simulink model "VehicleBackKin"  (R2024b)
settings: Solver=FixedStepAuto  StartTime=0.0  StopTime=inf  FixedStep=VehicleEnv.Ts  RelTol=1e-3
values from neighbouring files (symbols this model uses):
  em = ElectricMotor    [VehicleBackKinEnv.m]
  ess = VehicleEnv.ess    [VehicleBackKinEnv.m]
  fd = FinalDrive    [VehicleBackKinEnv.m]
  gb = Gearbox    [VehicleBackKinEnv.m]
  ice = Engine    [VehicleBackKinEnv.m]
  reward = VehicleEnv.reward    [VehicleBackKinEnv.m]
  selector_in = zeros(size(obs_info.Name))    [VehicleBackKinEnv.m]
  veh = Vehicle    [VehicleBackKinEnv.m]
  VehicleEnv = evalin("base","VehicleEnv")    [VehicleBackKinEnv.m]
  wh = Wheels    [VehicleBackKinEnv.m]
undefined symbols (not defined in the file or in its folder): agentSampleTime, cycle_insimulink, cycleTime, transfer_fun_coeff
libraries: simulink x3, rllib x1, autolibsharedcoreengin x1
(part 1 of 4)
settings Model: PauseTimes=144  Creator=d043083  LastModifiedBy=d043083
settings SolverCC: ZeroCrossAlgorithm=Adaptive
settings DebuggingCC: IgnoredZcDiagnostic=none
settings RTWCC: GPUComputeCapability=3.5

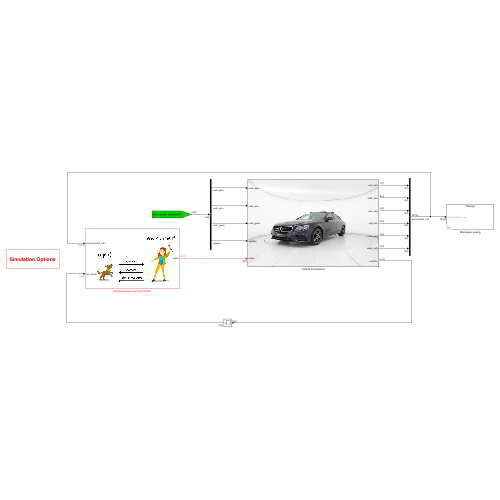
[thumbnail: Simulink's stored preview of the top-level diagram]
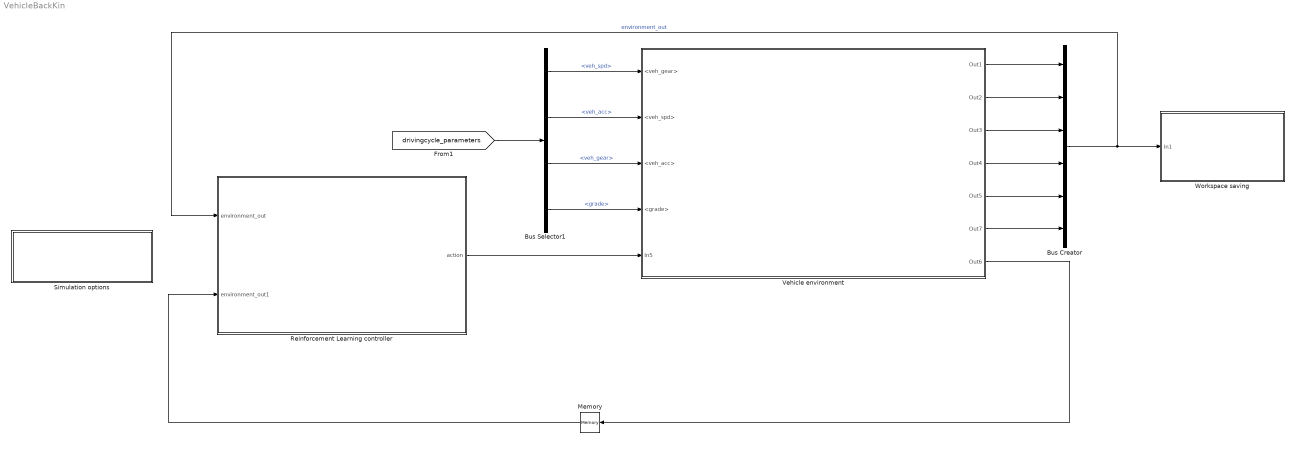
== system VehicleBackKin ==
  Bus Creator : BusCreator  Inputs=6
  Bus Selector1 : BusSelector  OutputSignals=veh_spd,veh_acc,veh_gear,grade
  Memory : Memory
  Reinforcement Learning controller : Subsystem
      mask Display: image('ReinforcementLearning.png'); % Use "Edit Image" on toolstrip to change.
  Simulation options : Subsystem  mask{veh_spd=cycle_insimulink.veh_spd, veh_gear=cycle_insimulink.veh_gear, veh_dist=cycle_insimulink.veh_dist, veh_dist_tot=cycle_insimulink.veh_dist.Data(end), grade=cycle_insimulink.grade}
      mask prompts: veh_spd "Vehicle speed array"; veh_gear "Vehicle gear array"; veh_dist "Vehicle distance array"; veh_dist_tot "Vehicle distance total"; grade "Grade array"
      mask Display: text(.5,.5,'\fontsize{20}{\bfSimulation Options}', 'hor','center','texmode','on');
  Vehicle environment : Subsystem
      mask Display: image('MercedesE.jpg'); % Use "Edit Image" on toolstrip to change.
  Workspace saving : Subsystem  Variant=on
  wires:
  [drivingcycle_parameters] -> Bus Selector1/1
  Bus Selector1/4 -> Vehicle environment/4(<grade>)  "<grade>"
  Bus Selector1/1 -> Vehicle environment/1(<veh_gear>)  "<veh_spd>"
  Bus Selector1/2 -> Vehicle environment/2(<veh_spd>)  "<veh_acc>"
  Bus Selector1/3 -> Vehicle environment/3(<veh_acc>)  "<veh_gear>"
  Vehicle environment/1(Out1) -> Bus Creator/1
  Vehicle environment/2(Out2) -> Bus Creator/2
  Vehicle environment/3(Out3) -> Bus Creator/3
  Vehicle environment/4(Out4) -> Bus Creator/4
  Vehicle environment/5(Out5) -> Bus Creator/5
  Reinforcement Learning controller/1(action) -> Vehicle environment/5(In5)
  Bus Creator/1 -> Reinforcement Learning controller/1(environment_out), Workspace saving/1(In1)  "environment_out"
  Vehicle environment/7(Out6) -> Memory/1
  Memory/1 -> Reinforcement Learning controller/2(environment_out1)
  Vehicle environment/6(Out7) -> Bus Creator/6

== system VehicleBackKin/Reinforcement Learning controller ==
  environment_out : Inport
  environment_out1 : Inport  Port=2
  Bus Selector : BusSelector  OutputSignals=ice_out.ice_bsfc,ice_out.ice_spd,batt_out.batt_pwr,batt_out.batt_soc,em_out.em_spd,gb_out.gb_in_spd,gb_out.gb_in_pwr
  Bus Selector2 : BusSelector  OutputSignals=veh_spd,veh_acc,veh_gear,grade,veh_dist,veh_dist_tot
  Bus Selector3 : BusSelector  OutputSignals=ice_out.ice_fuel_rate,batt_out.batt_soc,batt_out.batt_pwr
  Bus Selector4 : BusSelector  OutputSignals=batt_out.batt_soc
  Bus states : BusCreator  Inputs=12
  Divide : Product  Inputs=*/
  RL Agent : rllib/RL Agent  Agent=RLagent.agent  ExternalActionAsInput=off  ProvideLastAction=on  ProvideCumRwd=off  TreatAsDirectFeedthrough=on  UseStrictObservationDataTypes=off
  Reward : Subsystem  Variant=on
  Selector : Selector  InputPortWidth=12  IndexOptions=Index vector (port)  Indices=[1 2 3 4 5]  OutputSizes=1
  States normalization : MATLAB Function  TreatAsAtomicUnit=on  mask{states_max=VehicleEnv.normalization.states_max, states_min=VehicleEnv.normalization.states_min, upper=1, lower=0}
      mask prompts: states_max "Input max states vector"; states_min "Input min states vector"; upper "Input normalized max value"; lower "Input normalized min value"
  Transfer Fcn{1..5} (5 alike) : TransferFcn  Denominator=[transfer_fun_coeff 1]  ParameterTunability=Optimized
  agent_sampleTime : Constant  Value=agentSampleTime
  is_done : Subsystem
  selector_in : Constant  Value=selector_in
  action : Outport
  wires:
  Bus Selector3/2 -> Reward/2(batt_soc)  "<batt_soc>"
  [drivingcycle_parameters] -> Bus Selector2/1
  is_done/1(is_done) -> Reward/4(is_done), RL Agent/3
  Bus Selector4/1 -> is_done/1(environment_out)  "<batt_soc>"
  environment_out/1 -> Bus Selector4/1, Bus Selector3/1, Bus Selector/1
  Bus Selector3/3 -> Reward/3(batt_pwr)  "<batt_pwr>"
  Bus Selector3/1 -> Transfer Fcn1/1  "<ice_fuel_rate>"
  RL Agent/1 -> action/1  "action"
  Bus states/1 -> Selector/1
  States normalization/1(obs) -> RL Agent/1
  Bus Selector2/5 -> Divide/1  "<veh_dist>"
  Bus Selector2/6 -> Reward/7(veh_dist_tot), Divide/2  "<veh_dist_tot>"
  Bus Selector2/1 -> Bus states/1  "<veh_spd>"
  Bus Selector2/2 -> Bus states/2  "<veh_acc>"
  Bus Selector2/3 -> Bus states/3  "<veh_gear>"
  Bus Selector2/4 -> Bus states/4  "<grade>"
  Divide/1 -> Reward/6(veh_dist_perc), Bus states/5  "<veh_dist_perc>"
  Bus Selector/2 -> Transfer Fcn4/1  "<ice_spd>"
  Bus Selector/3 -> Transfer Fcn3/1  "<batt_pwr>"
  Bus Selector/4 -> Bus states/9  "<batt_soc>"
  Bus Selector/5 -> Bus states/10  "<em_spd>"
  Bus Selector/6 -> Bus states/11  "<gb_in_spd>"
  Bus Selector/7 -> Transfer Fcn2/1  "<gb_in_pwr>"
  Selector/1 -> States normalization/1(states)
  selector_in/1 -> Selector/2
  Transfer Fcn2/1 -> Bus states/12
  Transfer Fcn3/1 -> Bus states/8
  Transfer Fcn4/1 -> Bus states/7
  Reward/1(reward) -> RL Agent/2
  Transfer Fcn1/1 -> Reward/1(ice_fuel_rate)
  Bus Selector/1 -> Transfer Fcn5/1  "<ice_bsfc>"
  Transfer Fcn5/1 -> Bus states/6
  environment_out1/1 -> RL Agent/4  "last_action"
  agent_sampleTime/1 -> Reward/5(agent_sample_time)  "agent_sample_time"

== system VehicleBackKin/Simulation options ==
  Driving cycle parameters : Subsystem
  Vehicle parameters : Subsystem
  tag scope: drivingcycle_parameters=global, vehicle_parameters=global
  wires:
  Vehicle parameters/1(vehicle_parameters) -> [vehicle_parameters]
  Driving cycle parameters/1(Out1) -> [drivingcycle_parameters]

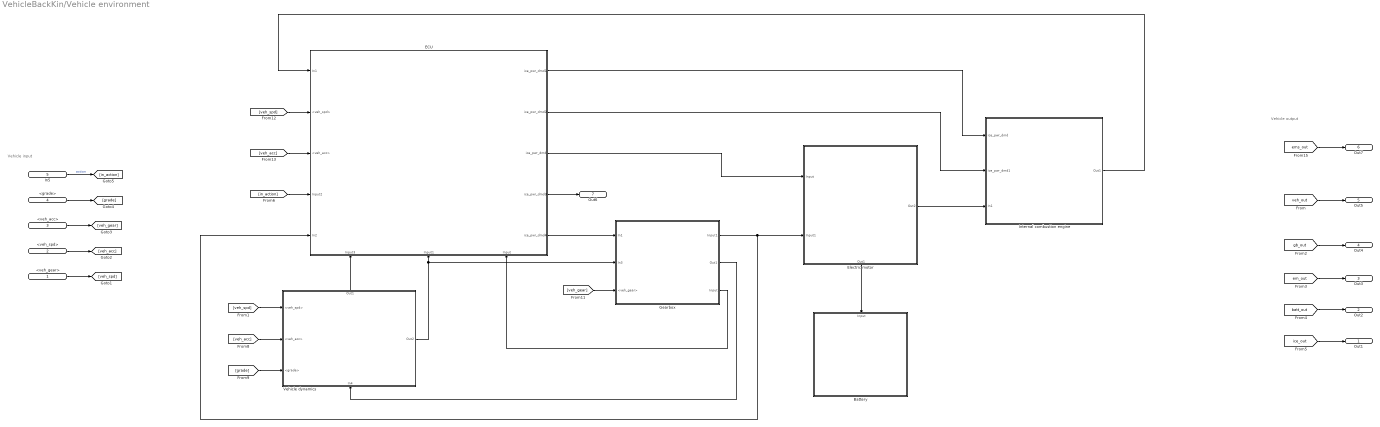
== system VehicleBackKin/Vehicle environment ==
  note: Vehicle input
  note: Vehicle output
  <veh_gear> : Inport
  <veh_spd> : Inport  Port=2
  <veh_acc> : Inport  Port=3
  <grade> : Inport  Port=4
  In5 : Inport  Port=5
  Battery : Subsystem
      settings: PortSchema="{\"entries\":[{\"content\":{\"sides\":[{\"content\":{},\"type\":\"ConnectorPlacement.EquallySpacedRectSide\",\"uuid\":\"5cc14c93-2257-4c42-96d2-5f70254acb0b\"},{\"content\":{\"side\":\"RIGHT\"},\"type\":\"ConnectorPlacement.EquallySpacedRectSide\",\"uuid\":\"885c1069-ef23-4d30-974e-45d76434d7c4\"},{\"content\":{\"side\":\"TOP\"},\"type\":\"ConnectorPlacement.EquallySpacedRectSide\",\"uuid\":\"ec9ecdea-bd65-4eb5-8cea-e0c874968461\"},{\"content\":{\"connectorIds\":[\"In1\"],\"side\":\"BOTTOM\"},\"type\":\"ConnectorPlacement.EquallySpacedRectSide\",\"uuid\":\"48f3ae7f-793f-4dcd-9fa1-914ff6f14037\"}]},\"type\":\"ConnectorPlacement.EquallySpacedConnector\",\"uuid\":\"1aa20074-a035-4ee9-ada4-5158e380f169\"}],\"packageUris\":[\"http://schema.mathworks.com/mf0/Connector/R2020b\"],\"version\":\"1.0\"}"
      mask Display: image('Batteria.jpg'); % Use "Edit Image" on toolstrip to change.
  ECU : Subsystem
      settings: PortSchema="{\"entries\":[{\"content\":{\"sides\":[{\"content\":{\"connectorIds\":[\"In1\",\"In2\",\"In3\",\"In4\",\"In5\"]},\"type\":\"ConnectorPlacement.EquallySpacedRectSide\",\"uuid\":\"6915b64d-6ea9-4067-95ac-c20354703ee7\"},{\"content\":{\"connectorIds\":[\"Out1\",\"Out2\",\"Out3\",\"Out4\",\"Out5\"],\"side\":\"RIGHT\"},\"type\":\"ConnectorPlacement.EquallySpacedRectSide\",\"uuid\":\"cf3d86e8-25dc-4d48-8f0f-305411c61d4f\"},{\"content\":{\"side\":\"TOP\"},\"type\":\"ConnectorPlacement.EquallySpacedRectSide\",\"uuid\":\"b1f23bea-e512-42b5-b538-919416972c81\"},{\"content\":{\"connectorIds\":[\"In6\",\"In7\",\"In8\"],\"side\":\"BOTTOM\"},\"type\":\"ConnectorPlacement.EquallySpacedRectSide\",\"uuid\":\"50fad9bb-c4f2-4285-a950-a1133b9213d3\"}]},\"type\":\"ConnectorPlacement.EquallySpacedConnector\",\"uuid\":\"19750d56-6156-4ef9-9a7b-4edf450523ed\"}],\"packageUris\":[\"http://schema.mathworks.com/mf0/Connector/R2020b\"],\"version\":\"1.0\"}"
      mask Display: image('Controllore.jpg'); % Use "Edit Image" on toolstrip to change.
  Electric motor : Subsystem
      settings: PortSchema="{\"entries\":[{\"content\":{\"sides\":[{\"content\":{\"connectorIds\":[\"In1\",\"In2\"]},\"type\":\"ConnectorPlacement.EquallySpacedRectSide\",\"uuid\":\"4621f324-a3a7-4840-813d-e50e1f5ceb3f\"},{\"content\":{\"connectorIds\":[\"Out1\"],\"side\":\"RIGHT\"},\"type\":\"ConnectorPlacement.EquallySpacedRectSide\",\"uuid\":\"633019f1-7db7-4c47-9c41-8b5307cf44fe\"},{\"content\":{\"connectorIds\":[\"Out2\"],\"side\":\"TOP\"},\"type\":\"ConnectorPlacement.EquallySpacedRectSide\",\"uuid\":\"d44403c4-92f8-40a4-ab8f-212953f0ff24\"},{\"content\":{\"side\":\"BOTTOM\"},\"type\":\"ConnectorPlacement.EquallySpacedRectSide\",\"uuid\":\"fcac849e-b2bd-4cc9-9f90-6c89c81f4505\"}]},\"type\":\"ConnectorPlacement.EquallySpacedConnector\",\"uuid\":\"caf37530-7cb9-457e-a5a4-eeae52c30c66\"}],\"packageUris\":[\"http://schema.mathworks.com/mf0/Connector/R2020b\"],\"version\":\"1.0\"}"
      mask Display: image('EM.jpg'); % Use "Edit Image" on toolstrip to change.
  Gearbox : Subsystem
      mask Display: image('AMT.jpg'); % Use "Edit Image" on toolstrip to change.
  Internal combustion engine : Subsystem
      mask Display: image('Engine.jpg'); % Use "Edit Image" on toolstrip to change.
  Vehicle dynamics : Subsystem
      settings: PortSchema="{\"entries\":[{\"content\":{\"sides\":[{\"content\":{\"connectorIds\":[\"In1\",\"In2\",\"In3\"]},\"type\":\"ConnectorPlacement.EquallySpacedRectSide\",\"uuid\":\"365e0bac-1e24-479d-b147-a682ee541f38\"},{\"content\":{\"connectorIds\":[\"Out1\"],\"side\":\"RIGHT\"},\"type\":\"ConnectorPlacement.EquallySpacedRectSide\",\"uuid\":\"2cbf8c85-0052-4455-b732-b9757e72a38e\"},{\"content\":{\"connectorIds\":[\"Out2\"],\"side\":\"TOP\"},\"type\":\"ConnectorPlacement.EquallySpacedRectSide\",\"uuid\":\"4b24f042-0800-48a3-9d68-f5545f81db88\"},{\"content\":{\"connectorIds\":[\"In4\"],\"side\":\"BOTTOM\"},\"type\":\"ConnectorPlacement.EquallySpacedRectSide\",\"uuid\":\"a2eac2b0-6dc4-4918-baf0-35537435d2ce\"}]},\"type\":\"ConnectorPlacement.EquallySpacedConnector\",\"uuid\":\"636e98cf-f787-478e-9789-5dec5969cd2f\"}],\"packageUris\":[\"http://schema.mathworks.com/mf0/Connector/R2020b\"],\"version\":\"1.0\"}"
      mask Display: image('MercedesE.jpg'); % Use "Edit Image" on toolstrip to change.
  Out1 : Outport
  Out2 : Outport  Port=2
  Out3 : Outport  Port=3
  Out4 : Outport  Port=4
  Out5 : Outport  Port=5
  Out7 : Outport  Port=6
  Out6 : Outport  Port=7
  wires:
  Electric motor/1(Out2) -> Internal combustion engine/3(In1)
  Electric motor/2(Out1) -> Battery/1(Input)
  ECU/3(ice_pwr_dmd) -> Electric motor/2(Input)
  Gearbox/1(Input1) -> ECU/5(In2), Electric motor/1(Input1)
  ECU/2(ice_pwr_dmd2) -> Internal combustion engine/2(ice_pwr_dmd1)
  ECU/1(ice_pwr_dmd1) -> Internal combustion engine/1(ice_pwr_dmd)
  Gearbox/2(Out1) -> Vehicle dynamics/4(In4)
  Vehicle dynamics/1(Out2) -> ECU/7(Input1), Gearbox/2(In3)
  <veh_gear>/1 -> [veh_spd]
  <veh_spd>/1 -> [veh_acc]
  <veh_acc>/1 -> [veh_gear]
  <grade>/1 -> [grade]
  In5/1 -> [in_action]  "action"
  [veh_out] -> Out5/1
  [batt_out] -> Out2/1
  [ice_out] -> Out1/1
  [gb_out] -> Out4/1
  [em_out] -> Out3/1
  [veh_spd] -> Vehicle dynamics/1(<veh_spd>)
  [veh_acc] -> Vehicle dynamics/2(<veh_acc>)
  [grade] -> Vehicle dynamics/3(<grade>)
  [veh_gear] -> Gearbox/3(<veh_gear>)
  [ems_out] -> Out7/1
  Vehicle dynamics/2(Out1) -> ECU/6(Input3)
  [veh_spd] -> ECU/2(<veh_spd>)
  [veh_acc] -> ECU/3(<veh_acc>)
  [in_action] -> ECU/4(Input2)
  Gearbox/3(Input) -> ECU/8(Input)
  Internal combustion engine/1(Out1) -> ECU/1(In1)
  ECU/4(ice_pwr_dmd3) -> Out6/1
  ECU/5(ice_pwr_dmd4) -> Gearbox/1(In1)

== system VehicleBackKin/Workspace saving ==
  In1 : Inport
  Testing : Subsystem  VariantControl=do_training==false
  Training : Subsystem  VariantControl=do_training==true

== system VehicleBackKin/Reinforcement Learning controller/Reward ==
  ice_fuel_rate : Inport
  batt_soc : Inport  Port=2
  batt_pwr : Inport  Port=3
  is_done : Inport  Port=4
  agent_sample_time : Inport  Port=5
  veh_dist_perc : Inport  Port=6
  veh_dist_tot : Inport  Port=7
  Dense : Subsystem  VariantControl="reward.reward_type==\"Dense\""
  Dense_multicycle : Subsystem  VariantControl="reward.reward_type==\"Dense_multicycle\""
  ECMS : Subsystem  VariantControl="reward.reward_type==\"ECMS\""
  SOC_BC : Subsystem  VariantControl="reward.reward_type==\"SOC_BC\""
  Sparse : Subsystem  VariantControl="reward.reward_type==\"Sparse\""
  reward : Outport

== system VehicleBackKin/Reinforcement Learning controller/is_done ==
  environment_out : Inport
  Clock1 : Clock
  Constant2 : Constant  Value=cycleTime
  Constant3 : Constant  Value=ess.soc_high
  Constant4 : Constant  Value=ess.soc_low
  GreaterThan : RelationalOperator  OutDataTypeStr=boolean  RndMeth=Simplest  InputSameDT=off
  GreaterThan1 : RelationalOperator  OutDataTypeStr=boolean  RndMeth=Simplest  InputSameDT=off
  OR : Logic  Operator=OR  Inputs=3  IconShape=distinctive  AllPortsSameDT=off  OutDataTypeStr=boolean
  cycle_time_compare : RelationalOperator  Operator===  OutDataTypeStr=boolean  RndMeth=Simplest  InputSameDT=off
  is_done : Outport
  wires:
  environment_out/1 -> GreaterThan1/2, GreaterThan/1
  Clock1/1 -> cycle_time_compare/1
  GreaterThan1/1 -> OR/2
  Constant4/1 -> GreaterThan1/1
  Constant2/1 -> cycle_time_compare/2
  Constant3/1 -> GreaterThan/2
  OR/1 -> is_done/1  "is_done"
  GreaterThan/1 -> OR/3
  cycle_time_compare/1 -> OR/1

== system VehicleBackKin/Simulation options/Driving cycle parameters ==
  Bus Creator : BusCreator  Inputs=6
  Derivative : Derivative
  From Workspace : FromWorkspace  VariableName=veh_spd
  From Workspace1 : FromWorkspace  VariableName=veh_gear
  From Workspace2 : FromWorkspace  VariableName=veh_dist
  From Workspace3 : FromWorkspace  VariableName=grade
  veh_dist_tot : Constant  Value=veh_dist_tot
  Out1 : Outport
  wires:
  Bus Creator/1 -> Out1/1  "driving_cycle"
  veh_dist_tot/1 -> Bus Creator/6  "veh_dist_tot"
  Derivative/1 -> Bus Creator/2  "veh_acc"
  From Workspace/1 -> Derivative/1, Bus Creator/1  "veh_spd"
  From Workspace1/1 -> Bus Creator/3  "veh_gear"
  From Workspace2/1 -> Bus Creator/4  "veh_dist"
  From Workspace3/1 -> Bus Creator/5  "grade"

== system VehicleBackKin/Simulation options/Vehicle parameters ==
  Battery parameters : Subsystem
  Bus Creator : BusCreator  Inputs=7
  EM parameters : Subsystem
  Final drive parameters : Subsystem
  Gearbox parameters : Subsystem
  ICE parameters : Subsystem
  Vehicle paramateres : Subsystem
  Wheels parameters : Subsystem
  vehicle_parameters : Outport
  wires:
  EM parameters/1(Out1) -> Bus Creator/5
  Final drive parameters/1(Out1) -> Bus Creator/3
  Battery parameters/1(Out1) -> Bus Creator/6
  Wheels parameters/1(Out1) -> Bus Creator/2
  ICE parameters/1(Out1) -> Bus Creator/7
  Vehicle paramateres/1(veh) -> Bus Creator/1
  Gearbox parameters/1(Out1) -> Bus Creator/4
  Bus Creator/1 -> vehicle_parameters/1  "vehicle_parameters"

== system VehicleBackKin/Vehicle environment/Battery ==
  note: Cell battery power
  Input : Inport
  Add : Sum
  Bus Creator : BusCreator  Inputs=4
  Cell current calculation : Subsystem
  Constant : Constant  Value=ess.accelec
  Constant1 : Constant  Value=ess.num_cell
  Constant2 : Constant  Value=ess.cell_cap
  Coulomb counting method : Subsystem
  Divide : Product  Inputs=*/
  tag scope: batt_out=global
  wires:
  Input/1 -> Add/1  "em_pwr_ele"
  Constant/1 -> Add/2
  Add/1 -> [batt_pwr], Divide/1  "batt_pwr"
  Constant1/1 -> Divide/2
  Divide/1 -> Cell current calculation/1(<cell_voc>1)  "battc_pwr"
  Cell current calculation/1(Out1) -> [battc_curr], Coulomb counting method/1(In1)
  Coulomb counting method/1(Out1) -> Cell current calculation/2(In4), Bus Creator/1
  Bus Creator/1 -> [batt_out]  "batt_out"
  [battc_curr] -> Bus Creator/4  "battc_curr"
  Cell current calculation/2(Out2) -> [battc_R]
  Cell current calculation/3(Out3) -> [battc_voc]
  Coulomb counting method/2(Out2) -> Bus Creator/2
  [batt_pwr] -> Bus Creator/3  "batt_pwr"
  Constant2/1 -> Coulomb counting method/2(<cell_cap>)

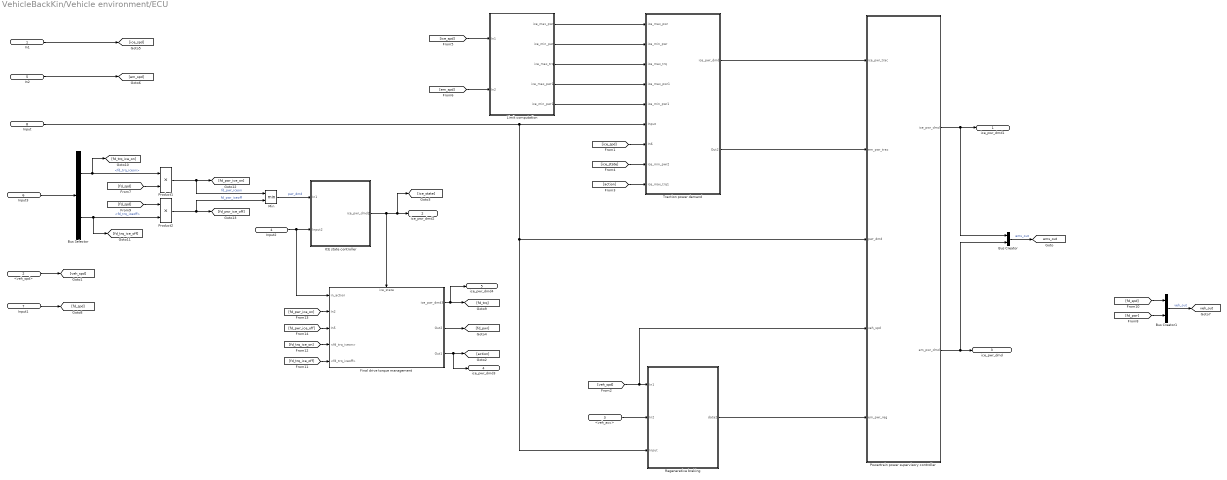
== system VehicleBackKin/Vehicle environment/ECU ==
  In1 : Inport
  <veh_spd> : Inport  Port=2
  <veh_acc> : Inport  Port=3
  Input2 : Inport  Port=4
  In2 : Inport  Port=5
  Input3 : Inport  Port=6
  Input1 : Inport  Port=7
  Input : Inport  Port=8
  Bus Creator : BusCreator  Inputs=2
  Bus Creator1 : BusCreator  Inputs=2
  Bus Selector : BusSelector  OutputSignals=fd_trq_iceon,fd_trq_iceoff
  Final drive torque management : Subsystem
      settings: PortSchema="{\"entries\":[{\"content\":{\"sides\":[{\"content\":{\"connectorIds\":[\"In1\",\"In2\",\"In3\",\"In4\",\"In5\"]},\"type\":\"ConnectorPlacement.EquallySpacedRectSide\",\"uuid\":\"c7a87722-dc4e-477a-be39-eaa96eedece7\"},{\"content\":{\"connectorIds\":[\"Out1\",\"Out2\",\"Out3\"],\"side\":\"RIGHT\"},\"type\":\"ConnectorPlacement.EquallySpacedRectSide\",\"uuid\":\"10d41276-04d9-41db-90f5-599bb14a1653\"},{\"content\":{\"connectorIds\":[\"In6\"],\"side\":\"TOP\"},\"type\":\"ConnectorPlacement.EquallySpacedRectSide\",\"uuid\":\"9a9e13cd-cff5-4257-9201-ca6e5cd22e86\"},{\"content\":{\"side\":\"BOTTOM\"},\"type\":\"ConnectorPlacement.EquallySpacedRectSide\",\"uuid\":\"fe064079-6754-4589-9e86-1f5b669b2d17\"}]},\"type\":\"ConnectorPlacement.EquallySpacedConnector\",\"uuid\":\"519b2432-dc70-4d8f-ad9c-aef518082c1b\"}],\"packageUris\":[\"http://schema.mathworks.com/mf0/Connector/R2020b\"],\"version\":\"1.0\"}"
  ICE state controller : Subsystem
  Limit computation : Subsystem
  Min : MinMax  Inputs=2
  Powertrain power supervisory controller : Stateflow chart  TreatAsAtomicUnit=on
  Product1 : Product
  Product2 : Product
  Regenerative braking : Subsystem
  Traction power demand : Subsystem
  ice_pwr_dmd1 : Outport
  ice_pwr_dmd2 : Outport  Port=2
  ice_pwr_dmd : Outport  Port=3
  ice_pwr_dmd3 : Outport  Port=4
  ice_pwr_dmd4 : Outport  Port=5
  tag scope: ems_out=global, veh_out=global
  wires:
  Limit computation/1(ice_max_pwr) -> Traction power demand/1(ice_max_pwr)
  Limit computation/5(ice_min_pwr1) -> Traction power demand/5(ice_min_pwr1)
  Limit computation/4(ice_max_pwr1) -> Traction power demand/4(ice_max_pwr1)
  Limit computation/3(ice_max_trq) -> Traction power demand/3(ice_max_trq)
  Limit computation/2(ice_min_pwr) -> Traction power demand/2(ice_min_pwr)
  In1/1 -> [ice_spd]
  In2/1 -> [em_spd]
  [ice_spd] -> Limit computation/1(In1)
  [em_spd] -> Limit computation/2(In2)
  Input/1 -> Regenerative braking/3(Input), Powertrain power supervisory controller/3(pwr_dmd), Traction power demand/6(Input)
  [veh_spd] -> Powertrain power supervisory controller/4(veh_spd), Regenerative braking/1(In1)
  <veh_acc>/1 -> Regenerative braking/2(In2)
  [ice_spd] -> Traction power demand/7(In6)
  Traction power demand/1(ice_pwr_dmd) -> Powertrain power supervisory controller/1(ice_pwr_trac)
  Traction power demand/2(Out2) -> Powertrain power supervisory controller/2(em_pwr_trac)
  Regenerative braking/1(data2) -> Powertrain power supervisory controller/5(em_pwr_reg)
  Powertrain power supervisory controller/1(ice_pwr_dmd) -> Bus Creator/1, ice_pwr_dmd1/1
  Powertrain power supervisory controller/2(em_pwr_dmd) -> Bus Creator/2, ice_pwr_dmd/1
  [ice_state] -> Traction power demand/8(ice_min_pwr2)
  [action] -> Traction power demand/9(ice_max_trq1)
  Bus Creator/1 -> [ems_out]  "ems_out"
  <veh_spd>/1 -> [veh_spd]
  ? -> ?
  ? -> ?
  [fd_pwr] -> Bus Creator1/2
  Bus Creator1/1 -> [veh_out]  "veh_out"
  Input1/1 -> [fd_spd]
  Input3/1 -> Bus Selector/1
  Bus Selector/1 -> Product1/1, [fd_trq_ice_on]  "<fd_trq_iceon>"
  [fd_spd] -> Product1/2
  Bus Selector/2 -> Product2/2, [fd_trq_ice_off]  "<fd_trq_iceoff>"
  [fd_spd] -> Bus Creator1/1
  Min/1 -> ICE state controller/1(In1)  "pwr_dmd"
  Input2/1 -> Final drive torque management/1(in_action), ICE state controller/2(Input2)
  ICE state controller/1(ice_pwr_dmd2) -> [ice_state], ice_pwr_dmd2/1, Final drive torque management/6(ice_state)
  Final drive torque management/2(Out2) -> [fd_pwr]
  Final drive torque management/1(ice_pwr_dmd3) -> ice_pwr_dmd4/1, [fd_trq]
  Final drive torque management/3(Out1) -> [action], ice_pwr_dmd3/1
  [fd_trq_ice_off] -> Final drive torque management/5(<fd_trq_iceoff>)
  [fd_trq_ice_on] -> Final drive torque management/4(<fd_trq_iceon>)
  [fd_spd] -> Product2/1
  Product1/1 -> Min/1, [fd_pwr_ice_on]  "fd_pwr_iceon"
  Product2/1 -> Min/2, [fd_pwr_ice_off]  "fd_pwr_iceoff"
  [fd_pwr_ice_on] -> Final drive torque management/2(In2)
  [fd_pwr_ice_off] -> Final drive torque management/3(In5)

== system VehicleBackKin/Vehicle environment/Electric motor ==
  note: EM efficiency
  note: EM electrical power
  note: EM speed
  Input1 : Inport
  Input : Inport  Port=2
  Bus Creator : BusCreator  Inputs=2
  Constant : Constant  Value=em.gear_ratio
  Divide : Product  Inputs=*/
  EffPwrMap : Lookup_n-D  BreakpointsForDimension1=em.EffPwrMap.brkp2  BreakpointsForDimension2=em.EffPwrMap.brkp1  Table=em.EffPwrMap.tab_data  InternalRulePriority=Speed  RndMeth=Simplest
      settings: InputPortMap=u0,u1
  Product : Product
  Product1 : Product
  Switch : Switch  Criteria=u2 > Threshold  SaturateOnIntegerOverflow=off  InputSameDT=off
  Out2 : Outport
  Out1 : Outport  Port=2
  tag scope: em_out=global
  wires:
  Input/1 -> [em_pwr], Product1/2, Divide/1, Switch/2, EffPwrMap/1  "em_pwr_dmd"
  Input1/1 -> Product/1  "gb_in_spd"
  Product/1 -> EffPwrMap/2, [em_spd]  "em_spd"
  EffPwrMap/1 -> Divide/2, Product1/1  "em_eff"
  Product1/1 -> Switch/3
  Divide/1 -> Switch/1
  Switch/1 -> Out1/1  "em_pwr_ele"
  [em_spd] -> Bus Creator/1
  [em_pwr] -> Bus Creator/2
  Bus Creator/1 -> [em_out]  "em_out"
  [em_spd] -> Out2/1
  Constant/1 -> Product/2

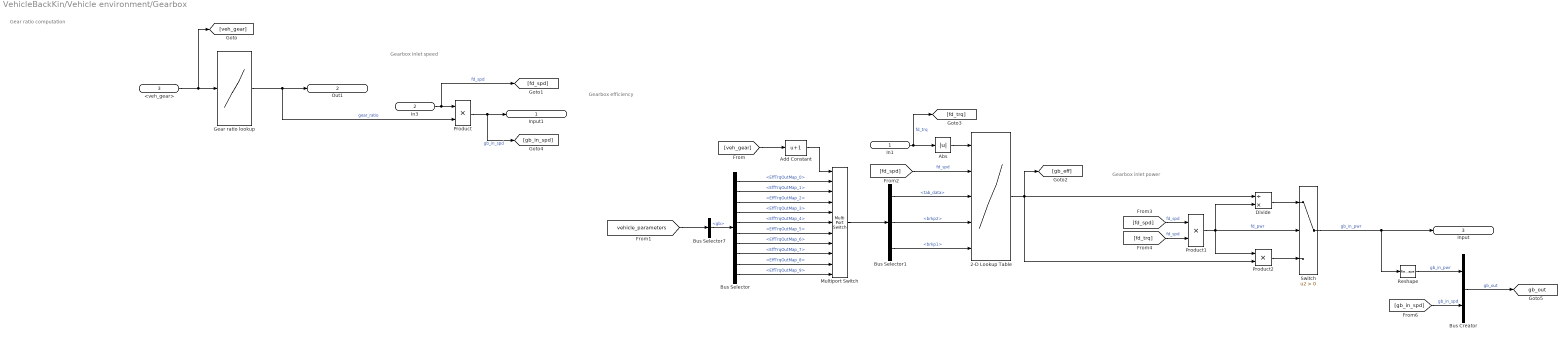
== system VehicleBackKin/Vehicle environment/Gearbox ==
  note: Gearbox inlet speed
  note: Gear ratio computation
  note: Gearbox efficiency
  note: Gearbox inlet power
  In1 : Inport
  In3 : Inport  Port=2
  <veh_gear> : Inport  Port=3
  2-D Lookup Table : Lookup_n-D  BreakpointsForDimension1Source=Input port  BreakpointsForDimension1=[1:3]  BreakpointsForDimension2Source=Input port  BreakpointsForDimension2=[1:3]  TableSource=Input port  InternalRulePriority=Speed  RndMeth=Simplest
      settings: InputPortMap=u0,u1,p221,p5,p7
  Abs : Abs  SaturateOnIntegerOverflow=off
  Add Constant : Bias  Bias=1  SaturateOnIntegerOverflow=off
  Bus Creator : BusCreator  Inputs=2
  Bus Selector : BusSelector  OutputSignals=EffTrqOutMap.EffTrqOutMap_0,EffTrqOutMap.EffTrqOutMap_1,EffTrqOutMap.EffTrqOutMap_2,EffTrqOutMap.EffTrqOutMap_3,EffTrqOutMap.EffTrqOutMap_4,EffTrqOutMap.EffTrqOutMap_5,EffTrqOutMap.EffTrqOutMap_6,EffTrqOutMap.EffTrqOutMap_7,EffTrqOutMap.EffTrqOutMap_8,EffTrqOutMap.EffTrqOutMap_9
  Bus Selector1 : BusSelector  OutputSignals=tab_data,brkp2,brkp1
  Bus Selector7 : BusSelector  OutputSignals=gb
  Divide : Product  Inputs=/*
  Gear ratio lookup : Lookup_n-D  NumberOfTableDimensions=1  BreakpointsForDimension1=gb.gear_idx  Table=gb.gear_ratio  InterpMethod=Flat  ExtrapMethod=Clip  InternalRulePriority=Speed  OutDataTypeStr=double  RndMeth=Simplest
  Multiport Switch : MultiPortSwitch  Inputs=10  SaturateOnIntegerOverflow=off  InputSameDT=off
  Product : Product
  Product1 : Product
  Product2 : Product
  Reshape : Reshape
  Switch : Switch  Criteria=u2 > Threshold  SaturateOnIntegerOverflow=off  InputSameDT=off
  Input1 : Outport
  Out1 : Outport  Port=2
  Input : Outport  Port=3
  tag scope: gb_out=global
  wires:
  Bus Selector/5 -> Multiport Switch/6  "<EffTrqOutMap_4>"
  Add Constant/1 -> Multiport Switch/1
  Bus Selector/1 -> Multiport Switch/2  "<EffTrqOutMap_0>"
  Bus Selector/2 -> Multiport Switch/3  "<EffTrqOutMap_1>"
  Bus Selector/3 -> Multiport Switch/4  "<EffTrqOutMap_2>"
  [vehicle_parameters] -> Bus Selector7/1
  Bus Selector/4 -> Multiport Switch/5  "<EffTrqOutMap_3>"
  Bus Selector/6 -> Multiport Switch/7  "<EffTrqOutMap_5>"
  In1/1 -> [fd_trq], Abs/1  "fd_trq"
  Bus Selector/7 -> Multiport Switch/8  "<EffTrqOutMap_6>"
  Bus Selector/8 -> Multiport Switch/9  "<EffTrqOutMap_7>"
  Bus Selector/9 -> Multiport Switch/10  "<EffTrqOutMap_8>"
  Bus Selector/10 -> Multiport Switch/11  "<EffTrqOutMap_9>"
  Multiport Switch/1 -> Bus Selector1/1
  Abs/1 -> 2-D Lookup Table/1
  Bus Selector1/1 -> 2-D Lookup Table/3  "<tab_data>"
  Bus Selector1/2 -> 2-D Lookup Table/4  "<brkp2>"
  Bus Selector1/3 -> 2-D Lookup Table/5  "<brkp1>"
  Product/1 -> [gb_in_spd], Input1/1  "gb_in_spd"
  Bus Selector7/1 -> Bus Selector/1  "<gb>"
  <veh_gear>/1 -> [veh_gear], Gear ratio lookup/1
  Gear ratio lookup/1 -> Out1/1, Product/2  "gear_ratio"
  In3/1 -> [fd_spd], Product/1  "fd_spd"
  [veh_gear] -> Add Constant/1
  [fd_spd] -> 2-D Lookup Table/2  "fd_spd"
  [fd_spd] -> Product1/1  "fd_spd"
  [fd_trq] -> Product1/2  "fd_spd"
  Product1/1 -> Product2/1, Divide/2, Switch/2  "fd_pwr"
  Divide/1 -> Switch/1
  Product2/1 -> Switch/3
  Switch/1 -> Input/1, Reshape/1  "gb_in_pwr"
  [gb_in_spd] -> Bus Creator/2  "gb_in_spd"
  Bus Creator/1 -> [gb_out]  "gb_out"
  2-D Lookup Table/1 -> Divide/1, Product2/2, [gb_eff]
  Reshape/1 -> Bus Creator/1  "gb_in_pwr"
